simulink model "QBot2e_Workspace"  (R2020a)
settings: Solver=ode1  StartTime=0.0  StopTime=inf  FixedStep=1/250  RelTol=1e-3  EnableMultiTasking=on
model workspace (MAT data in the model file):
  cameraStepSize = Simulink.Parameter
  cameraStepSize.Value = Simulink.data.Expression
  cameraStepSize.Value.ExpressionString = "qc_get_step_size * ceil (1/30 /qc_get_step_size)"
  cameraStepSize.DataType = 'auto'
  cameraStepSize.Dimensions = -1
  internalStepSize = Simulink.Parameter
  internalStepSize.Value = Simulink.data.Expression
  internalStepSize.Value.ExpressionString = "qc_get_step_size * ceil(1/120 /qc_get_step_size)"
  internalStepSize.DataType = 'auto'
  internalStepSize.Dimensions = -1
  mainStepSize = Simulink.Parameter
  mainStepSize.Value = Simulink.data.Expression
  mainStepSize.Value.ExpressionString = "qc_get_step_size"
  mainStepSize.DataType = 'auto'
  mainStepSize.Dimensions = -1
undefined symbols (not defined in the file): qc_get_step_size
libraries: quarc_library x12, simulink_extras x2, simulink x2
settings Model: SimulationMode=external  ExtModeTrigDuration=10000  OrderedModelArguments=off  Creator=mbohra  LastModifiedBy=mbohra
settings SolverCC: PositivePriorityOrder=on
settings DataIOCC: SaveOutput=off  SignalLogging=off  DSMLogging=off  SaveTime=off  ReturnWorkspaceOutputs=off
settings DebuggingCC: ArithmeticOperatorsInVariantConditions=warning
settings SFSimCC: SimUseLocalCustomCode=off  CustomCodeUndefinedFunction=UseInterfaceOnly
settings RTWCC: Description=QUARC Win64 Target Using Toolchain  SystemTargetFile=quarc_win64.tlc  TemplateMakefile=quarc_default_tmf  RTWUseLocalCustomCode=off  Toolchain=QUARC win64 | nmake (64-bit Windows)  BuildConfiguration=Faster Runs
settings CodeAppCC: StateflowObjectComments=on
settings STFCustomTargetCC: TargetLangStandard=C99 (ISO)  ConcurrentExecutionCompliant=on  GRTInterface=on  UseToolchainInfoCompliant=on  SystemTargetFile=quarc_win64.tlc
settings GRTTargetCC: ParMdlRefBuildCompliant=off  CompOptLevelCompliant=off  CombineOutputUpdateFcns=off  MatFileLogging=off  CPPClassGenCompliant=off  GRTInterface=on  ExtMode=on  ExtModeMexFile=quarc_comm
settings ConfigComp: CovMetricSettings=dswe

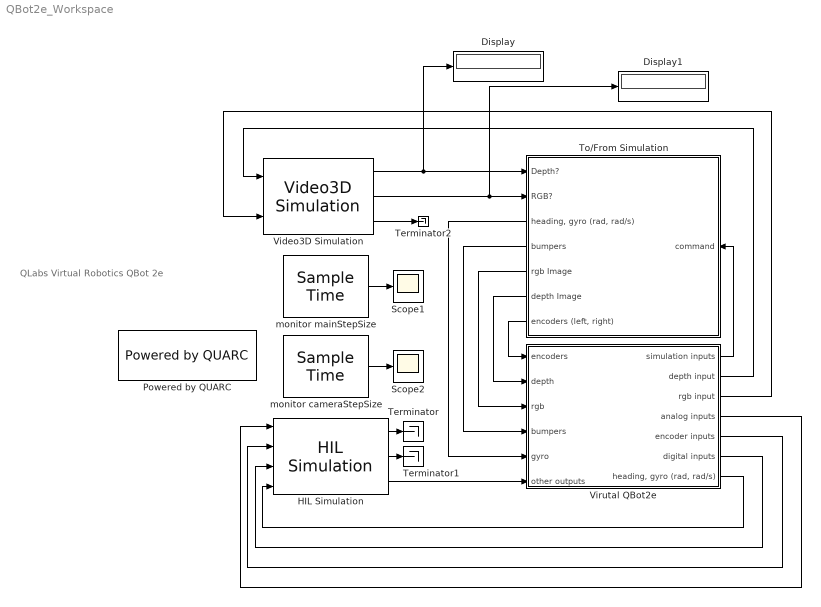
== system QBot2e_Workspace ==
  note: QLabs Virtual Robotics
      | QBot 2e
  Display : Display
  Display1 : Display
  HIL Simulation : quarc_library/Data Acquisition/Generic/Configuration/HIL Simulation  uri=tcpip://localhost:18910  board_type=qbot2e  board_id=0  sample_time=mainStepSize  active=on  num_clocks=1  num_interrupts=0  num_analog_inputs=1  num_analog_outputs=0  initial_analog=[]  num_digital_io=0  num_digital_inputs=59  num_digital_outputs=32  initial_digital=[]  num_encoder_inputs=2  num_pwm_outputs=2  initial_pwm=[]  other_inputs=[1002 3002]  other_outputs=[2000:2001 14000 16000]  initial_other=[]  integer_properties=[]  double_properties=[]  string_properties=[]
      settings: SourceProductName=QUARC Targets
  Powered by QUARC : quarc_library/Logos/Powered by QUARC
  Scope1 : Scope
  Scope2 : Scope
  Terminator : Terminator
  Terminator1 : Terminator
  Terminator2 : Terminator
  To/From Simulation : Subsystem
      settings: PortSchema="{\"entries\":[{\"content\":{\"sides\":[{\"content\":{\"connectorIds\":[\"In1\"]},\"type\":\"ConnectorPlacement.EquallySpacedRectSide\",\"uuid\":\"9c46811c-bdb3-4b06-a83d-707c145db3e3\"},{\"content\":{\"connectorIds\":[\"In2\",\"In3\",\"Out1\",\"Out2\",\"Out3\",\"Out4\",\"Out5\"],\"side\":\"RIGHT\"},\"type\":\"ConnectorPlacement.EquallySpacedRectSide\",\"uuid\":\"2e71cb5e-0160-4a21-8d6d-8c01db7ab905\"},{\"content\":{\"connectorIds\":[],\"side\":\"TOP\"},\"type\":\"ConnectorPlacement.EquallySpacedRectSide\",\"uuid\":\"db2307f6-be72-424f-9f3a-37d139d364ad\"}]},\"type\":\"ConnectorPlacement.EquallySpacedConnector\",\"uuid\":\"f65580c2-9ce9-4a50-a10c-6486b87fa517\"}],\"packageUris\":[\"http://schema.mathworks.com/mf0/Connector/19700101\"],\"version\":\"1.0\"}"
  Video3D Simulation : quarc_library/Multimedia/Video3D Simulation  uri=tcpip://localhost:18911  device_id=0  sample_time=cameraStepSize  show_in_use=on  active=on  depth_indices=[0]  depth_scales=9.44  depth_widths=[640]  depth_heights=[480]  depth_rates=[30]  rgb_indices=[0]  rgb_widths=[640]  rgb_heights=[480]  rgb_rates=[30]  infrared_indices=[]  infrared_widths=[640]  infrared_heights=[480]  infrared_rates=[90]  fisheye_indices=[]  fisheye_widths=[640]  fisheye_heights=[480]  fisheye_rates=[30]  gyro_indices=[]  accel_indices=[]  pose_indices=[]
      settings: SourceProductName=QUARC Targets
  Virutal QBot2e : Subsystem
  monitor cameraStepSize : quarc_library/Sources/Time/Sample Time  Priority=-99  sample_time=cameraStepSize
  monitor mainStepSize : quarc_library/Sources/Time/Sample Time  Priority=-99  sample_time=mainStepSize
  wires:
  monitor mainStepSize/1 -> Scope1/1
  HIL Simulation/3 -> Virutal QBot2e/6(other outputs)
  Virutal QBot2e/1(simulation inputs) -> To/From Simulation/1(command)
  To/From Simulation/3(rgb Image) -> Virutal QBot2e/3(rgb)
  To/From Simulation/4(depth Image) -> Virutal QBot2e/2(depth)
  Virutal QBot2e/4(analog inputs) -> HIL Simulation/1
  Virutal QBot2e/5(encoder inputs) -> HIL Simulation/2
  monitor cameraStepSize/1 -> Scope2/1
  Virutal QBot2e/3(rgb input) -> Video3D Simulation/2
  Virutal QBot2e/6(digital inputs) -> HIL Simulation/3
  To/From Simulation/2(bumpers) -> Virutal QBot2e/4(bumpers)
  To/From Simulation/1("heading, gyro (rad, rad/s)") -> Virutal QBot2e/5(gyro)
  Virutal QBot2e/7("heading, gyro (rad, rad/s)") -> HIL Simulation/4
  HIL Simulation/1 -> Terminator/1
  HIL Simulation/2 -> Terminator1/1
  Virutal QBot2e/2(depth input) -> Video3D Simulation/1
  To/From Simulation/5("encoders (left, right)") -> Virutal QBot2e/1(encoders)
  Video3D Simulation/3 -> Terminator2/1
  Video3D Simulation/1 -> Display/1, To/From Simulation/2(Depth?)
  Video3D Simulation/2 -> Display1/1, To/From Simulation/3(RGB?)

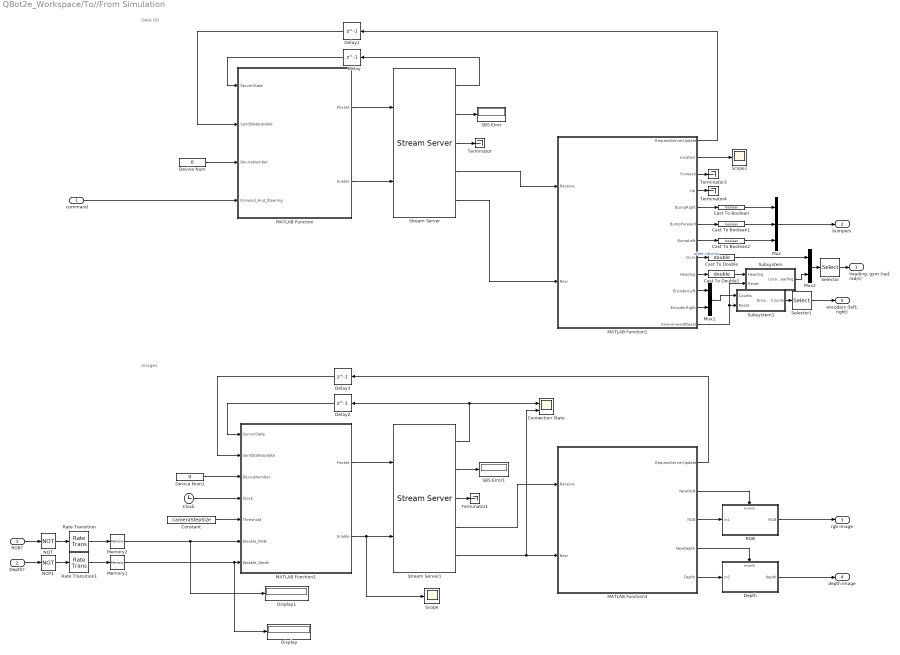
== system QBot2e_Workspace/To//From Simulation ==
  note: Images
  note: Data I/O
  command : Inport
  Depth? : Inport  Port=2
  RGB? : Inport  Port=3
  Cast To Boolean : DataTypeConversion  OutDataTypeStr=boolean
  Cast To Boolean1 : DataTypeConversion  OutDataTypeStr=boolean
  Cast To Boolean2 : DataTypeConversion  OutDataTypeStr=boolean
  Cast To Double : DataTypeConversion  OutDataTypeStr=double
  Cast To Double1 : DataTypeConversion  OutDataTypeStr=double
  Clock : Clock
  "Connection State " : Scope  NumInputPorts=2
  Constant : Constant  Value=cameraStepSize
  Delay : Delay  DelayLength=1
  Delay1 : Delay  DelayLength=1
  Delay2 : Delay  DelayLength=1  SampleTime=mainStepSize
  Delay3 : Delay  DelayLength=1  SampleTime=mainStepSize
  Depth : Subsystem
  Device Num : Constant  Value=0
  Device Num1 : Constant  Value=0  SampleTime=mainStepSize
  Display : Display
  Display1 : Display
  MATLAB Function : MATLAB Function  TreatAsAtomicUnit=on
  MATLAB Function1 : MATLAB Function  TreatAsAtomicUnit=on
  MATLAB Function2 : MATLAB Function  TreatAsAtomicUnit=on
  MATLAB Function3 : MATLAB Function  TreatAsAtomicUnit=on
  Memory1 : Memory  InitialCondition=1
  Memory2 : Memory  InitialCondition=1
  Mux : Mux  Inputs=3
  Mux1 : Mux  Inputs=2
  Mux2 : Mux  Inputs=2
  NOT : Logic  Operator=NOT  IconShape=distinctive  AllPortsSameDT=off  OutDataTypeStr=boolean
  NOT1 : Logic  Operator=NOT  IconShape=distinctive  AllPortsSameDT=off  OutDataTypeStr=boolean
  RGB : Subsystem
  Rate Transition : RateTransition
  Rate Transition1 : RateTransition
  SBS Error : Display
  SBS Error1 : Display
  Scope : Scope
  Scope1 : Scope
  Selector : Selector  InputPortWidth=2  IndexOptions=Index vector (dialog)  Indices=[2 1]  OutputSizes=1
  Selector1 : Selector  InputPortWidth=2  IndexOptions=Index vector (dialog)  Indices=[2 1]  OutputSizes=1
  Stream Server : quarc_library/Communications/Basic/Stream Server  uri_source=Specify via dialog (do not evaluate)  uri=tcpip://remotehost:18001?nagle='off'  apply_uri_to_all_configs=on  send_buffer_size=65537  receive_buffer_size=65537  byte_order=little endian (Intel - LSB first)  optimization=Minimum latency  send_options=Send all data  receive_options=Receive all data  default_value=[0]  sample_time=qc_get_step_size  active=on  implementation=Use blocking I/O in a separate thread  send_fifo_size=3  receive_fifo_size=3  send_priority=0  receive_priority=0  send_dimensions=on  receive_dimensions=on  max_dimensions=65537  data_type=uint8  type_expr=BusObject
      settings: AttributesFormatString="\"tcpip://remotehost:18001?nagle='off'\""
  Stream Server1 : quarc_library/Communications/Basic/Stream Server  uri_source=Specify via dialog (do not evaluate)  uri=tcpip://remotehost:18002?nagle='off'  apply_uri_to_all_configs=on  send_buffer_size=65537  receive_buffer_size=100000  byte_order=little endian (Intel - LSB first)  optimization=Minimum latency  send_options=Send all data  receive_options=Receive all data  default_value=[0]  sample_time=mainStepSize  active=on  implementation=Use blocking I/O in a separate thread  send_fifo_size=3  receive_fifo_size=1  send_priority=0  receive_priority=0  send_dimensions=on  receive_dimensions=on  max_dimensions=65537  data_type=uint8  type_expr=BusObject
      settings: AttributesFormatString="\"tcpip://remotehost:18002?nagle='off'\""
  Subsystem : Subsystem
  Subsystem1 : Subsystem
  Terminator{,1,3..4} (4 alike) : Terminator
  "heading, gyro (rad, rad/s)" : Outport
  bumpers : Outport  Port=2
  rgb Image : Outport  Port=3
  depth Image : Outport  Port=4
  "encoders (left, right)" : Outport  Port=5
  wires:
  MATLAB Function1/1(RequestServerUpdate) -> Delay1/1
  Stream Server/1 -> Delay/1
  Delay1/1 -> MATLAB Function/2(SendStateUpdate)
  Stream Server/3 -> Terminator/1
  Stream Server/2 -> SBS Error/1
  Stream Server/5 -> MATLAB Function1/2(New)
  MATLAB Function/2(Enable) -> Stream Server/2
  Device Num/1 -> MATLAB Function/3(DeviceNumber)
  MATLAB Function/1(Packet) -> Stream Server/1
  Stream Server/4 -> MATLAB Function1/1(Receive)
  Delay/1 -> MATLAB Function/1(ServerState)
  MATLAB Function1/2(Location) -> Scope1/1
  Stream Server1/1 -> "Connection State "/1, Delay2/1
  Delay2/1 -> MATLAB Function2/1(ServerState)
  Delay3/1 -> MATLAB Function2/2(SendStateUpdate)
  MATLAB Function2/1(Packet) -> Stream Server1/1
  MATLAB Function2/2(Enable) -> Scope/1, Stream Server1/2
  Device Num1/1 -> MATLAB Function2/3(DeviceNumber)
  Stream Server1/2 -> SBS Error1/1
  Stream Server1/3 -> Terminator1/1
  Stream Server1/5 -> "Connection State "/2, MATLAB Function3/2(New)
  Stream Server1/4 -> MATLAB Function3/1(Receive)
  MATLAB Function3/1(RequestServerUpdate) -> Delay3/1
  MATLAB Function1/8(Gyro) -> Cast To Double/1  "other returns"
  Mux/1 -> bumpers/1
  MATLAB Function1/5(BumpRight) -> Cast To Boolean/1
  MATLAB Function1/6(BumpForward) -> Cast To Boolean1/1
  MATLAB Function1/7(BumpLeft) -> Cast To Boolean2/1
  Cast To Boolean/1 -> Mux/1
  Cast To Boolean1/1 -> Mux/2
  Cast To Boolean2/1 -> Mux/3
  Cast To Double/1 -> Mux2/1
  MATLAB Function1/3(Forward) -> Terminator3/1
  MATLAB Function1/4(Up) -> Terminator4/1
  MATLAB Function3/4(NewDepth) -> Depth/Enable
  MATLAB Function3/2(NewRGB) -> RGB/Enable
  Depth/1(depth) -> depth Image/1
  RGB/1(RGB) -> rgb Image/1
  MATLAB Function3/3(RGB) -> RGB/1(In1)
  MATLAB Function3/5(Depth) -> Depth/1(In1)
  Clock/1 -> MATLAB Function2/4(Clock)
  Constant/1 -> MATLAB Function2/5(Threshold)
  command/1 -> MATLAB Function/4(Forward_And_Steering)
  MATLAB Function1/10(EncoderLeft) -> Mux1/1
  MATLAB Function1/11(EncoderRight) -> Mux1/2
  Mux1/1 -> Subsystem1/1(Counts)
  MATLAB Function1/9(Heading) -> Cast To Double1/1
  Mux2/1 -> Selector/1
  Selector/1 -> "heading, gyro (rad, rad/s)"/1
  Cast To Double1/1 -> Subsystem/1(Heading)
  Subsystem/1(Local Heading) -> Mux2/2
  MATLAB Function1/12(EnvironmentReset) -> Subsystem1/2(Reset), Subsystem/2(Reset)
  Selector1/1 -> "encoders (left, right)"/1
  Subsystem1/1(Encoder Counts) -> Selector1/1
  RGB?/1 -> NOT/1
  Rate Transition1/1 -> Memory1/1
  NOT1/1 -> Rate Transition1/1
  Depth?/1 -> NOT1/1
  Rate Transition/1 -> Memory2/1
  NOT/1 -> Rate Transition/1
  Memory2/1 -> Display1/1, MATLAB Function2/6(Disable_RGB)
  Memory1/1 -> Display/1, MATLAB Function2/7(Disable_Depth)

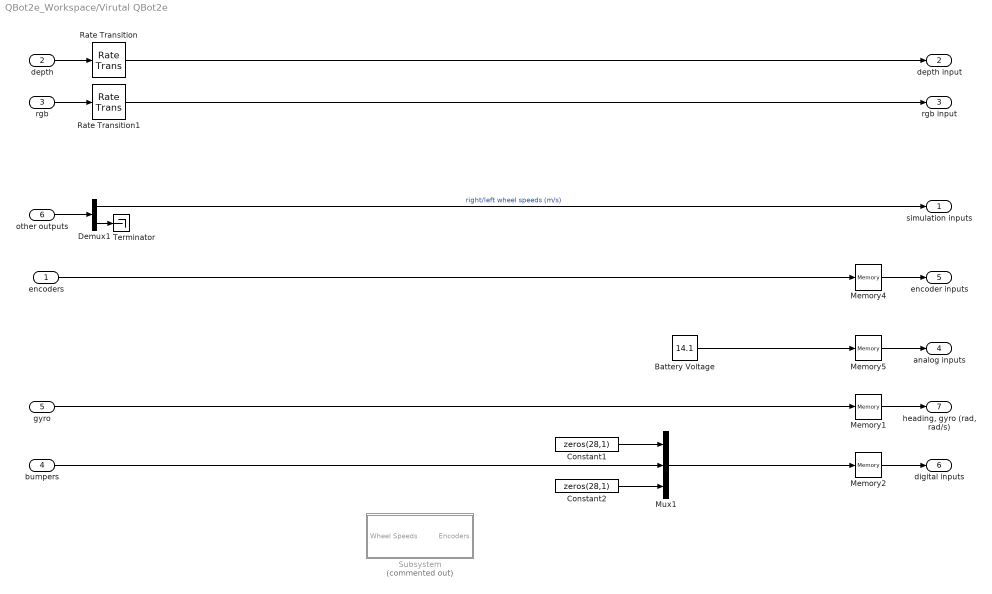
== system QBot2e_Workspace/Virutal QBot2e ==
  encoders : Inport
  depth : Inport  Port=2
  rgb : Inport  Port=3
  bumpers : Inport  Port=4
  gyro : Inport  Port=5
  other outputs : Inport  Port=6
  Battery Voltage : Constant  Value=14.1
  Constant1 : Constant  Value=zeros(28,1)  OutDataTypeStr=boolean
  Constant2 : Constant  Value=zeros(28,1)  OutDataTypeStr=boolean
  Demux1 : Demux  Outputs=[2 2]
  Memory1 : Memory
  Memory2 : Memory  InitialCondition=zeros(59,1)
  Memory4 : Memory  InitialCondition=[0 0]
  Memory5 : Memory
  Mux1 : Mux  Inputs=3
  Rate Transition : RateTransition
  Rate Transition1 : RateTransition
  Subsystem : Subsystem  Commented=on
  Terminator : Terminator
  simulation inputs : Outport
  depth input : Outport  Port=2  VectorParamsAs1DForOutWhenUnconnected=off
  rgb input : Outport  Port=3  VectorParamsAs1DForOutWhenUnconnected=off
  analog inputs : Outport  Port=4
  encoder inputs : Outport  Port=5
  digital inputs : Outport  Port=6  VectorParamsAs1DForOutWhenUnconnected=off
  "heading, gyro (rad, rad/s)" : Outport  Port=7
  wires:
  Memory4/1 -> encoder inputs/1
  Demux1/1 -> simulation inputs/1  "right/left wheel speeds (m/s)"
  Memory5/1 -> analog inputs/1
  Battery Voltage/1 -> Memory5/1
  Constant1/1 -> Mux1/1
  Mux1/1 -> Memory2/1
  bumpers/1 -> Mux1/2
  depth/1 -> Rate Transition/1
  rgb/1 -> Rate Transition1/1
  gyro/1 -> Memory1/1
  Memory1/1 -> "heading, gyro (rad, rad/s)"/1
  Memory2/1 -> digital inputs/1
  Constant2/1 -> Mux1/3
  other outputs/1 -> Demux1/1
  Demux1/2 -> Terminator/1
  Rate Transition/1 -> depth input/1
  Rate Transition1/1 -> rgb input/1
  encoders/1 -> Memory4/1

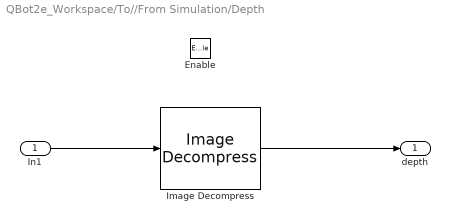
== system QBot2e_Workspace/To//From Simulation/Depth ==
  In1 : Inport
  Enable : EnablePort
  Image Decompress : quarc_library/Image Processing/Generic/Image Decompress  algorithm=JPEG  resolution=640 x 480  width=640  height=480  output_format=MATLAB RGB (HxWx3)  data_type=uint8
      settings: AttributesFormatString=(%<algorithm>)  SourceProductName=QUARC Targets
  depth : Outport  VectorParamsAs1DForOutWhenUnconnected=off
  wires:
  Image Decompress/1 -> depth/1
  In1/1 -> Image Decompress/1

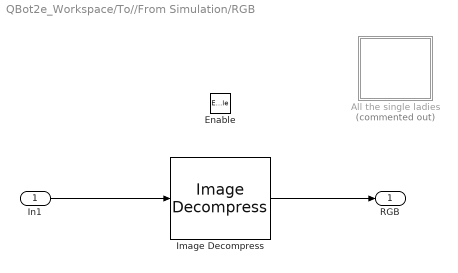
== system QBot2e_Workspace/To//From Simulation/RGB ==
  In1 : Inport
  Enable : EnablePort
  All the single ladies : Subsystem  Commented=on
  Image Decompress : quarc_library/Image Processing/Generic/Image Decompress  algorithm=JPEG  resolution=640 x 480  width=640  height=480  output_format=MATLAB RGB (HxWx3)  data_type=uint8
      settings: AttributesFormatString=(%<algorithm>)  SourceProductName=QUARC Targets
  RGB : Outport  VectorParamsAs1DForOutWhenUnconnected=off
  wires:
  In1/1 -> Image Decompress/1
  Image Decompress/1 -> RGB/1

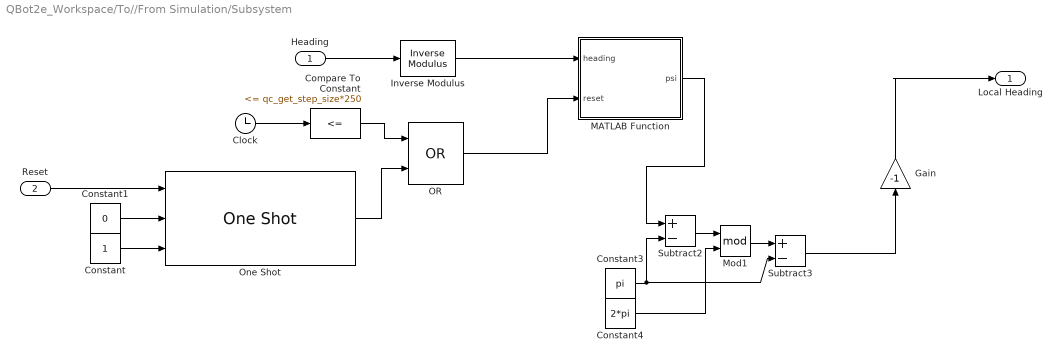
== system QBot2e_Workspace/To//From Simulation/Subsystem ==
  Heading : Inport
  Reset : Inport  Port=2
  Clock : Clock
  Compare To Constant : simulink/Logic and Bit Operations/Compare To Constant  relop=<=  const=qc_get_step_size*250  OutDataTypeStr=boolean
  Constant : Constant
  Constant1 : Constant  Value=0
  Constant3 : Constant  Value=pi
  Constant4 : Constant  Value=2*pi
  Gain : Gain  Gain=-1
  Inverse Modulus : quarc_library/Discontinuities/Inverse Modulus  modulus=2*pi  output_derivative=off  output_revolutions=off  max_x=Inf  min_x=-Inf
  MATLAB Function : MATLAB Function  TreatAsAtomicUnit=on
  Mod1 : Math  Operator=mod  SignedPower=on  SaturateOnIntegerOverflow=on
  OR : Logic  Operator=OR  IconShape=distinctive  AllPortsSameDT=off  OutDataTypeStr=boolean
  One Shot : quarc_library/Discontinuities/One Shot  trigger_type=Rising edge  redun_pulse=Ignore extraneous pulse  width_source=Specify via dialog  pulse_width=250
      settings: SourceProductName=QUARC Targets
  Subtract2 : Sum  Inputs=+-
  Subtract3 : Sum  Inputs=+-
  Local Heading : Outport  VectorParamsAs1DForOutWhenUnconnected=off
  wires:
  Heading/1 -> Inverse Modulus/1
  Inverse Modulus/1 -> MATLAB Function/1(heading)
  Reset/1 -> One Shot/1
  OR/1 -> MATLAB Function/2(reset)
  Clock/1 -> Compare To Constant/1
  Compare To Constant/1 -> OR/1
  One Shot/1 -> OR/2
  Constant/1 -> One Shot/3
  Constant1/1 -> One Shot/2
  Subtract2/1 -> Mod1/1
  Constant4/1 -> Mod1/2
  Constant3/1 -> Subtract3/2, Subtract2/2
  Mod1/1 -> Subtract3/1
  MATLAB Function/1(psi) -> Subtract2/1
  Subtract3/1 -> Gain/1
  Gain/1 -> Local Heading/1

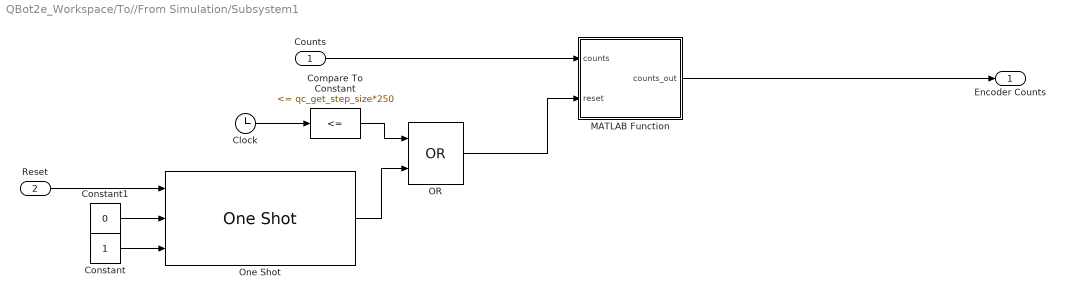
== system QBot2e_Workspace/To//From Simulation/Subsystem1 ==
  Counts : Inport
  Reset : Inport  Port=2
  Clock : Clock
  Compare To Constant : simulink/Logic and Bit Operations/Compare To Constant  relop=<=  const=qc_get_step_size*250  OutDataTypeStr=boolean
  Constant : Constant
  Constant1 : Constant  Value=0
  MATLAB Function : MATLAB Function  TreatAsAtomicUnit=on
  OR : Logic  Operator=OR  IconShape=distinctive  AllPortsSameDT=off  OutDataTypeStr=boolean
  One Shot : quarc_library/Discontinuities/One Shot  trigger_type=Rising edge  redun_pulse=Ignore extraneous pulse  width_source=Specify via dialog  pulse_width=250
      settings: SourceProductName=QUARC Targets
  Encoder Counts : Outport  VectorParamsAs1DForOutWhenUnconnected=off
  wires:
  Counts/1 -> MATLAB Function/1(counts)
  Reset/1 -> One Shot/1
  OR/1 -> MATLAB Function/2(reset)
  Clock/1 -> Compare To Constant/1
  Compare To Constant/1 -> OR/1
  One Shot/1 -> OR/2
  Constant/1 -> One Shot/3
  Constant1/1 -> One Shot/2
  MATLAB Function/1(counts_out) -> Encoder Counts/1

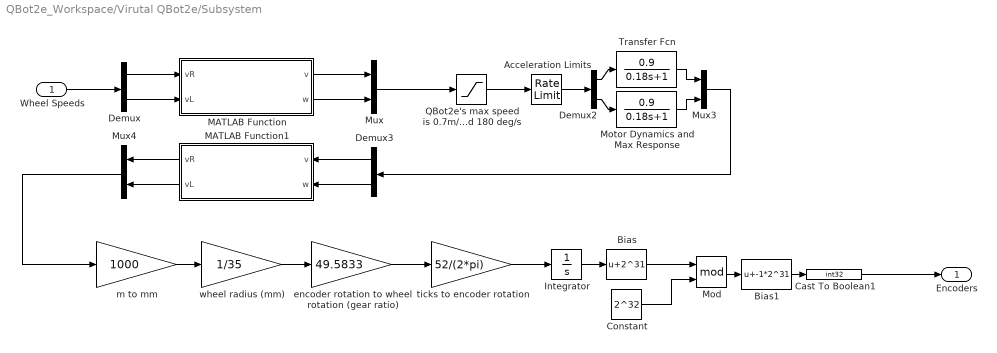
== system QBot2e_Workspace/Virutal QBot2e/Subsystem ==
  Wheel Speeds : Inport
  " encoder rotation to wheel rotation (gear ratio)" : Gain  Gain=49.5833
  Acceleration Limits : RateLimiter  RisingSlewLimit=[5 40]  FallingSlewLimit=-1*[5 40]  SampleTimeMode=inherited
  Bias : Bias  Bias=2^31
  Bias1 : Bias  Bias=-1*2^31
  Cast To Boolean1 : DataTypeConversion  OutDataTypeStr=int32
  Constant : Constant  Value=2^32
  Demux : Demux  Outputs=2
  Demux2 : Demux  Outputs=2
  Demux3 : Demux  Outputs=2
  Integrator : Integrator
  MATLAB Function : MATLAB Function  TreatAsAtomicUnit=on
  MATLAB Function1 : MATLAB Function  TreatAsAtomicUnit=on
  Mod : Math  Operator=mod  SignedPower=on  SaturateOnIntegerOverflow=on
  Motor Dynamics and Max Response : TransferFcn  Numerator=[0.9]  Denominator=[0.18 1]
  Mux : Mux  Inputs=2
  Mux3 : Mux  Inputs=2
  Mux4 : Mux  Inputs=2
  QBot2e's max speed is 0.7m/s and 180 deg/s : Saturate  UpperLimit=[0.7 pi]  LowerLimit=-1*[0.7 pi]
  Transfer Fcn : TransferFcn  Numerator=[0.9]  Denominator=[0.18 1]
  m to mm : Gain  Gain=1000
  ticks to encoder rotation : Gain  Gain=52/(2*pi)
  wheel radius (mm) : Gain  Gain=1/35
  Encoders : Outport  VectorParamsAs1DForOutWhenUnconnected=off
  wires:
  ticks to encoder rotation/1 -> Integrator/1
  Mod/1 -> Bias1/1
  Cast To Boolean1/1 -> Encoders/1
  Bias/1 -> Mod/1
  MATLAB Function/1(v) -> Mux/1
  m to mm/1 -> wheel radius (mm)/1
  Constant/1 -> Mod/2
  wheel radius (mm)/1 -> " encoder rotation to wheel rotation (gear ratio)"/1
  MATLAB Function/2(w) -> Mux/2
  Demux/1 -> MATLAB Function/1(vR)
  Integrator/1 -> Bias/1
  Mux/1 -> QBot2e's max speed is 0.7m/s and 180 deg/s/1
  Demux/2 -> MATLAB Function/2(vL)
  Bias1/1 -> Cast To Boolean1/1
  MATLAB Function1/2(vL) -> Mux4/2
  " encoder rotation to wheel rotation (gear ratio)"/1 -> ticks to encoder rotation/1
  Demux3/2 -> MATLAB Function1/2(w)
  Demux2/2 -> Motor Dynamics and Max Response/1
  Motor Dynamics and Max Response/1 -> Mux3/2
  MATLAB Function1/1(vR) -> Mux4/1
  Mux4/1 -> m to mm/1
  QBot2e's max speed is 0.7m/s and 180 deg/s/1 -> Acceleration Limits/1
  Transfer Fcn/1 -> Mux3/1
  Demux2/1 -> Transfer Fcn/1
  Acceleration Limits/1 -> Demux2/1
  Mux3/1 -> Demux3/1
  Demux3/1 -> MATLAB Function1/1(v)
  Wheel Speeds/1 -> Demux/1

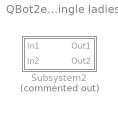
== system QBot2e_Workspace/To//From Simulation/RGB/All the single ladies ==
  Subsystem2 : Subsystem  Commented=on

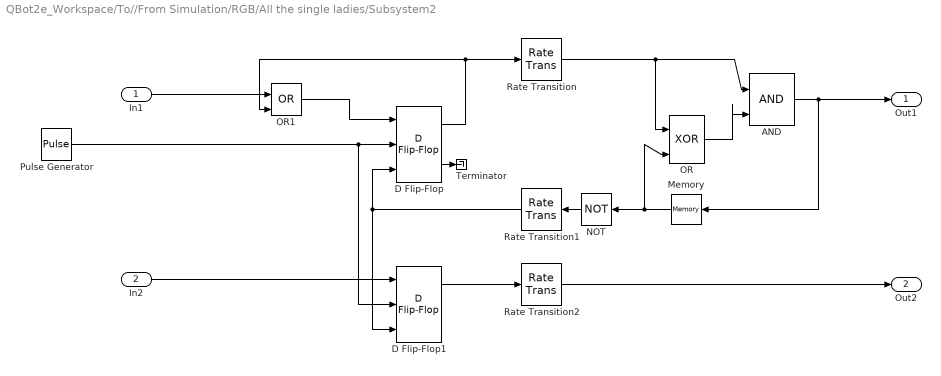
== system QBot2e_Workspace/To//From Simulation/RGB/All the single ladies/Subsystem2 ==
  In1 : Inport
  In2 : Inport  Port=2
  AND : Logic  IconShape=distinctive  AllPortsSameDT=off  OutDataTypeStr=boolean
  D Flip-Flop : simulink_extras/Flip Flops/D Flip-Flop
  D Flip-Flop1 : simulink_extras/Flip Flops/D Flip-Flop
  Memory : Memory  InheritSampleTime=on
  NOT : Logic  Operator=NOT  IconShape=distinctive  AllPortsSameDT=off  OutDataTypeStr=boolean
  OR : Logic  Operator=XOR  IconShape=distinctive  AllPortsSameDT=off  OutDataTypeStr=boolean
  OR1 : Logic  Operator=OR  IconShape=distinctive  AllPortsSameDT=off  OutDataTypeStr=boolean
  Pulse Generator : DiscretePulseGenerator  PulseType=Time based  Period=0.002  PulseWidth=50
  Rate Transition : RateTransition  OutPortSampleTime=internalStepSize
  Rate Transition1 : RateTransition
  Rate Transition2 : RateTransition  OutPortSampleTime=internalStepSize
  Terminator : Terminator
  Out1 : Outport  VectorParamsAs1DForOutWhenUnconnected=off
  Out2 : Outport  Port=2  VectorParamsAs1DForOutWhenUnconnected=off
  wires:
  AND/1 -> Memory/1, Out1/1
  OR/1 -> AND/2
  Memory/1 -> NOT/1, OR/2
  In1/1 -> OR1/1
  Pulse Generator/1 -> D Flip-Flop1/2, D Flip-Flop/2
  D Flip-Flop/1 -> OR1/2, Rate Transition/1
  Rate Transition/1 -> AND/1, OR/1
  OR1/1 -> D Flip-Flop/1
  Rate Transition1/1 -> D Flip-Flop/3, D Flip-Flop1/3
  NOT/1 -> Rate Transition1/1
  D Flip-Flop/2 -> Terminator/1
  In2/1 -> D Flip-Flop1/1
  D Flip-Flop1/1 -> Rate Transition2/1
  Rate Transition2/1 -> Out2/1

== matlab function QBot2e_Workspace/To//From Simulation/Subsystem1/MATLAB Function ==
  data: counts input; counts_out output; reset input
function counts_out = fcn(counts, reset)

persistent counts_offset
if isempty(counts_offset)
    counts_offset = counts;
end

if reset 
    counts_offset = counts;
end

counts_out = counts - counts_offset;

== matlab function QBot2e_Workspace/To//From Simulation/MATLAB Function1 ==
  data: Receive input size=65537; RequestServerUpdate output; New input; Location output; Forward output; Up output; BumpRight output; BumpForward output; BumpLeft output; Gyro output; Heading output; EncoderLeft output; EncoderRight output; EnvironmentReset output
function [RequestServerUpdate, Location, Forward, Up, BumpRight, BumpForward, BumpLeft, Gyro, Heading, EncoderLeft, EncoderRight, EnvironmentReset]  = QBotApplicationWorkspaceDecodeDataPacket(Receive, New)

%% Setup

persistent iLocation;
persistent iForward;
persistent iUp;
persistent iBumpForward;
persistent iBumpLeft;
persistent iBumpRight;
persistent iGyro;
persistent iHeading;
persistent iEncoderLeft;
persistent iEncoderRight;

if isempty(iLocation)
    iLocation = [single(0); single(0); single(0)];
    iForward = [single(0); single(0); single(0)];
    iUp = [single(0); single(0); single(0)];
    iBumpForward = uint8(0);
    iBumpLeft = uint8(0);
    iBumpRight = uint8(0);
    iGyro = single(0);
    iHeading = single(0);
    iEncoderLeft = int32(0);
    iEncoderRight = int32(0);
end

% Need to assign outputs here even though they are reassigned at the end
% since matlab can't determine the signal widths
Location = [single(0); single(0); single(0)];
Forward = [single(0); single(0); single(0)];
Up = [single(0); single(0); single(0)];
BumpForward = uint8(0);
BumpLeft = uint8(0);
BumpRight = uint8(0);
Gyro = single(0);
EnvironmentReset = 0;
Heading = single(0);
EncoderLeft = int32(0);
EncoderRight = int32(0);

RequestServerUpdate = 0;
PacketSize = length(Receive);

% Packet > 0, new data, and magic number in first index
if ((PacketSize > 0) && (New == 1) && (Receive(1) == uint8(123)))
    
    %skip magic number
    Index = int32(2);
    
    while(Index <= PacketSize)
       
        %% Get container details
        ContainerSize = typecast(uint8(flip(Receive(Index:Index+3))), 'int32');
        DeviceID = typecast(uint8(flip(Receive(Index+4:Index+7))), 'int32');
        DeviceNum = typecast(uint8(flip(Receive(Index+8:Index+11))), 'int32');
        DeviceFunction = uint8(Receive(Index+12));
        PayloadStart = Index+13;
        PayloadEnd = Index+ContainerSize-1;
        
        %% Pass container to appropriate decoding function
        if (DeviceID == 20) %is this a QBot container?
            
            if (DeviceFunction == 11) %UE4 State Response
                [iLocation, iForward, iUp, iBumpForward, iBumpLeft, iBumpRight, iGyro, iHeading, iEncoderLeft, iEncoderRight] = QBot2eDecodeUE4StateContainer(Receive, PayloadStart);
                RequestServerUpdate = 1;
            end
        
        elseif (DeviceID == 1001) %Simulink notification
            if (DeviceFunction == 200) %Reset button
                EnvironmentReset = 1;
            end
        end
        
        
        
        %% Process next container if any data is left.
        Index = Index+ContainerSize;
    end


end

Location = iLocation;
Forward = iForward;
Up = iUp;
BumpForward = iBumpForward;
BumpLeft = iBumpLeft;
BumpRight = iBumpRight;
Gyro = iGyro;
Heading = iHeading;
EncoderLeft = iEncoderLeft;
EncoderRight = iEncoderRight;

== matlab function QBot2e_Workspace/To//From Simulation/MATLAB Function ==
  settings: updateMethod=DISCRETE  sampleTime=qc_get_step_size
  data: Packet output size=65537; ServerState input; SendStateUpdate input; Enable output; DeviceNumber input; Forward_And_Steering input
function [Packet,Enable] = QBotApplicationWorkspaceMakePacketData(ServerState, SendStateUpdate, DeviceNumber, Forward_And_Steering) 

% Be sure to set the maximum signal size of the variable size Packet port 
% in Simulink->Edit Data of the editor window.  Size should be 65537 or
% larger to ensure that the stream server generates a 4 byte packet size.

%% Setup
persistent LastServerState;

if isempty(LastServerState)
    LastServerState = uint8(0);
end

Enable = 0;
Packet = uint8([]);

%% On connection
if ((ServerState == 2) && (LastServerState ~= 2))
    Packet = QBot2eMakeCommandStateContainer(DeviceNumber, Forward_And_Steering(1), Forward_And_Steering(2));
end

%% Send new State Container
% Previous state processed, send a new one
if (SendStateUpdate)
    Packet = QBot2eMakeCommandStateContainer(DeviceNumber, Forward_And_Steering(1), Forward_And_Steering(2));
end

%% Transmit
% If we have data to send, enable the transmit
PacketLength = length(Packet);

if (PacketLength > 0)
    % Add magic byte.  This is just for error handling and isn't typically
    % required in simulink, but useful in lower-level languages like Python
    Packet = [uint8(123); Packet];
    
    Enable = 1; 
end


LastServerState = ServerState;

== matlab function QBot2e_Workspace/Virutal QBot2e/Subsystem/MATLAB Function ==
  data: vR input; v output; vL input; w output
function [v, w] = qBotForKin(vR, vL)

d = 0.235; % meters
v = (vR + vL)/2;
w = (vR - vL)/d;

== matlab function QBot2e_Workspace/To//From Simulation/MATLAB Function2 ==
  settings: updateMethod=DISCRETE  sampleTime=mainStepSize
  data: Packet output size=65537; ServerState input; SendStateUpdate input; Enable output; DeviceNumber input; Clock input; Threshold input; Disable_RGB input; Disable_Depth input
function [Packet,Enable] = QBotApplicationWorkspaceMakeVideoPacketData(ServerState, SendStateUpdate, DeviceNumber, Clock, Threshold, Disable_RGB, Disable_Depth) 

% Be sure to set the maximum signal size of the variable size Packet port 
% in Simulink->Edit Data of the editor window.  Size should be 65537 or
% larger to ensure that the stream server generates a 4 byte packet size.

%% Setup
persistent LastServerState;
persistent timeLastSend;
persistent readyToSend;

if isempty(LastServerState)
    LastServerState = uint8(0);
    readyToSend = uint8(0);
    timeLastSend = -Threshold;
end

Enable = 0;
Packet = uint8([]);

%% On connection
if ((ServerState == 2) && (LastServerState ~= 2))
    if (Disable_RGB == 0)
        Packet = QBot2eMakeRGBRequestContainer(DeviceNumber);
    end
    
    if (Disable_Depth == 0)
        Packet = [Packet; QBot2eMakeDepthRequestContainer(DeviceNumber)];
    end
    
    if ((Disable_RGB == 1) && (Disable_Depth == 1))
        % Do this to keep the server connection alive and avoid the
        % reconnection overhead
        Packet = QBot2eMakePingRequestContainer(DeviceNumber);
    end

end

% if ((ServerState == 2) && (LastServerState ~= 2))
%     Packet = QBot2eMakeRGBRequestContainer(DeviceNumber);
%     Packet = [Packet; QBot2eMakeDepthRequestContainer(DeviceNumber)];
% end

%% Send new State Container
% Previous state processed, send a new one
if (SendStateUpdate)
    readyToSend = uint8(1);
end

if readyToSend && (Clock - timeLastSend) > Threshold
    if (Disable_RGB == 0)
        Packet = QBot2eMakeRGBRequestContainer(DeviceNumber);
    end
    
    if (Disable_Depth == 0)
        Packet = [Packet; QBot2eMakeDepthRequestContainer(DeviceNumber)];
    end
    
    if ((Disable_RGB == 1) && (Disable_Depth == 1))
        % Do this to keep the server connection alive and avoid the
        % reconnection overhead
        Packet = QBot2eMakePingRequestContainer(DeviceNumber);
    end
%     Packet = QBot2eMakeRGBRequestContainer(DeviceNumber);
%     Packet = [Packet; QBot2eMakeDepthRequestContainer(DeviceNumber)];    
    readyToSend = uint8(0);
    timeLastSend = Clock;
end

%% Transmit
% If we have data to send, enable the transmit
PacketLength = length(Packet);

if (PacketLength > 0)
    % Add magic byte.  This is just for error handling and isn't typically
    % required in simulink, but useful in lower-level languages like Python
    Packet = [uint8(123); Packet];
    
    Enable = 1; 
end

LastServerState = ServerState;

== matlab function QBot2e_Workspace/To//From Simulation/MATLAB Function3 ==
  data: Receive input size=65537; RequestServerUpdate output; NewRGB output; New input; RGB output size=65537; NewDepth output; Depth output size=65537
function [RequestServerUpdate, NewRGB, RGB, NewDepth, Depth]  = QBotApplicationWorkspaceDecodeVideoPacket(Receive, New)

%% Setup

RGB = uint8([]);
Depth = uint8([]);

NewRGB = 0;
NewDepth = 0;

RequestServerUpdate = 0;
PacketSize = length(Receive);

% Packet > 0, new data, and magic number in first index
if ((PacketSize > 0) && (New == 1) && (Receive(1) == uint8(123)))
    
    %skip magic number
    Index = int32(2);
    
    while(Index <= PacketSize)
       
        %% Get container details
        ContainerSize = typecast(uint8(flip(Receive(Index:Index+3))), 'int32');
        DeviceID = typecast(uint8(flip(Receive(Index+4:Index+7))), 'int32');
        DeviceNum = typecast(uint8(flip(Receive(Index+8:Index+11))), 'int32');
        DeviceFunction = uint8(Receive(Index+12));
        PayloadStart = Index+13;
        PayloadEnd = Index+ContainerSize-1;
        
        %% Pass container to appropriate decoding function
        if (DeviceID == 20) %is this a QBot container?
            
            if (DeviceFunction == 101) % Pull out RGB payload for external processing
                RGBSize = typecast(uint8(flip(Receive(PayloadStart:PayloadStart+3))), 'int32');
                RGB = Receive(PayloadStart+4:PayloadEnd);
                NewRGB = 1;
                RequestServerUpdate = 1;
                
            elseif (DeviceFunction == 111) % Pull out Depth payload for external processing
                DepthSize = typecast(uint8(flip(Receive(PayloadStart:PayloadStart+3))), 'int32');
                Depth = Receive(PayloadStart+4:PayloadEnd);
                NewDepth = 1;
                RequestServerUpdate = 1;
            end
        end
        
        
        
        %% Process next container if any data is left.
        Index = Index+ContainerSize;
    end


end

== matlab function QBot2e_Workspace/Virutal QBot2e/Subsystem/MATLAB Function1 ==
  data: v input; vR output; w input; vL output
function [vR, vL] = qBotForKin(v, w)

d = 0.235; % meters
vR = v + d*w/2;
vL = v - d*w/2;

== matlab function QBot2e_Workspace/To//From Simulation/Subsystem/MATLAB Function ==
  data: heading input; psi output; reset input
function psi = fcn(heading, reset)

persistent heading_offset
if isempty(heading_offset)
    heading_offset = heading;
end

if reset 
    heading_offset = heading;
end

psi = heading - heading_offset;
% psi = mod(psi, 2*pi);
